simulink model "gm_sampleModel2049_sub"  (R2023a)
settings: Solver=VariableStepAuto  StartTime=0.0  StopTime=10.0  RelTol=1e-3
libraries: simulink x2, hdlsllib x1
settings Model: Creator=user1  LastModifiedBy=user1
settings OptimizationCC: BlockReduction=off  ConditionallyExecuteInputs=off
settings DebuggingCC: InheritedTsInSrcMsg=none

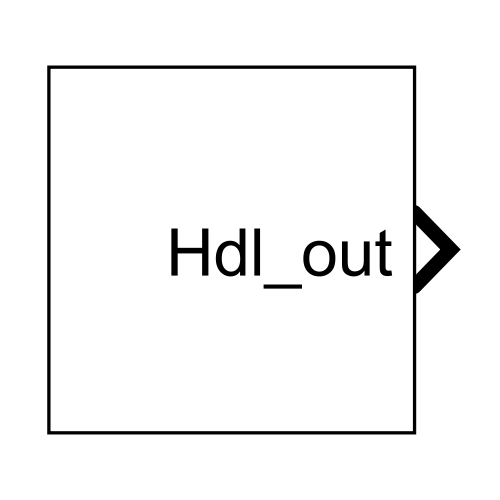
[thumbnail: Simulink's stored preview of the top-level diagram]
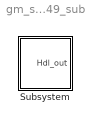
== system gm_sampleModel2049_sub ==
  Subsystem : Subsystem

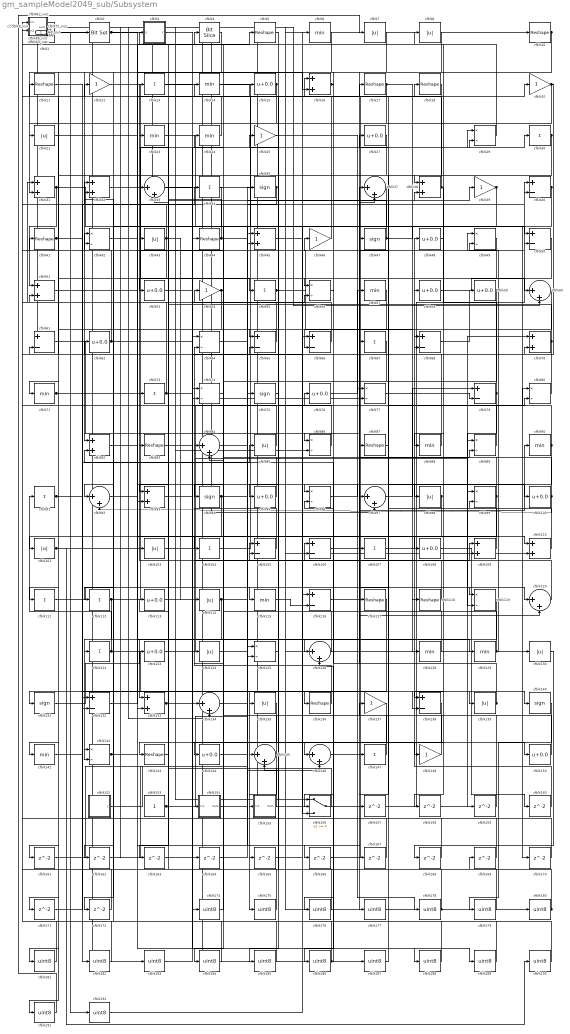
== system gm_sampleModel2049_sub/Subsystem ==
  cfblk1 : simulink/Logic and Bit Operations/Detect Increase  vinit=0.0  OutDataTypeStr=uint8
      settings: LibrarySourceBlock=|
      | hdlsllib/Logic and Bit
      | Operations/Detect
      | Increase
  cfblk{5,10..11,17..18,41,44,83,87,117..118,136,143} (13 alike) : Reshape
  cfblk{15,27,48,53,58..59,62,76,95,100,108,113,123,144,150} (15 alike) : Bias  Bias=0.0  SaturateOnIntegerOverflow=off
  cfblk{7..8,21,43,85,98,101,103,114,124,130,135,139} (13 alike) : Abs  OutDataTypeStr=uint8  SaturateOnIntegerOverflow=off
  cfblk102_inst : Subsystem
  cfblk{13,30,34,55,67,73,91,104,107,111..112,122,147} (13 alike) : Sum  Inputs=+  OutDataTypeStr=uint8
  cfblk{40,50,61,65..66,68,79,105..106,116,132,138} (12 alike) : Sum  Inputs=+-  OutDataTypeStr=uint8
  cfblk{16,31..32,38,45,51,70,82,93,109..110,133} (12 alike) : Sum  OutDataTypeStr=uint8
  cfblk{6,14,23..24,57,71,88,90,115,128..129,141} (12 alike) : MinMax  OutDataTypeStr=uint8
  cfblk{29,42,49,56,64,74,77,80,86,89,96,99,119,125,142} (15 alike) : Product  Inputs=*/  OutDataTypeStr=uint8  RndMeth=Zero  SaturateOnIntegerOverflow=on
  cfblk{12,20,25,39,46,54,137,148} (8 alike) : Gain  OutDataTypeStr=uint8
  cfblk{33,37,60,84,92,97,120,126,134,145..146} (11 alike) : Sum  Inputs=|++  OutDataTypeStr=uint8
  cfblk121_inst : Subsystem
  cfblk127_inst : Subsystem
  cfblk{35,47,75,94,131,140} (6 alike) : Signum
  cfblk152 : Subsystem  mask(Counter Free-Running){NumBits=double(16), tsamp=double(-1)}
      mask prompts: NumBits "Simulink:masks:NumberOfBits_MP"; tsamp "Simulink:masks:SampleTime_MP"
      mask help: Simulink:masks:CounterFreeRunning_MD
  cfblk153 : Constant  OutDataTypeStr=uint8  SampleTime=-1
  cfblk154 : Subsystem
  cfblk155 : Subsystem
  cfblk156 : Switch  OutDataTypeStr=uint8  SaturateOnIntegerOverflow=off  InputSameDT=off
  cfblk{157..172} (16 alike) : Delay  SampleTime=1
  cfblk{174..192} (19 alike) : DataTypeConversion  OutDataTypeStr=uint8  SaturateOnIntegerOverflow=off  RndMeth=Floor
  cfblk19_inst : Subsystem
  cfblk2 : simulink/Logic and Bit Operations/Bit Set  iBit=0
      settings: LibrarySourceBlock=|
      | hdlsllib/Logic and Bit
      | Operations/Bit Set
  cfblk26_inst : Subsystem
  cfblk28_inst : Subsystem
  cfblk3 : Subsystem  mask(Detect Rise Nonnegative){vinit=double(0), InputProcessing=Elements as channels (sample based), OutDataTypeStr=uint8}
      mask prompts: vinit "Simulink:masks:InitialCondition_MP"; InputProcessing "Simulink:masks:InputProcessing_MP"; OutDataTypeStr "Simulink:masks:OutputDataType_MP"
      mask help: Simulink:masks:DetectRiseNonnegative_MD
      mask init:
      | InputProcessing = 'Elements as channels (sample based)';
      | OutDataTypeStr = 'uint8';
      | vinit = double(0);
      mask TypeOptions InputProcessing: Simulink:masks:ColumnsAsChannelsFrameBased | Simulink:masks:ElementsAsChannelsSampleBased
      mask TypeOptions OutDataTypeStr: Simulink:masks:uint8 | Simulink:masks:boolean
      mask Display: fprintf('U >= 0\n&  NOT\nU/z >= 0')
  cfblk36_inst : Subsystem
  cfblk4 : hdlsllib/Logic and Bit Operations/Bit Slice  lidx=7  ridx=0
  cfblk63_inst : Subsystem
  cfblk69_inst : Subsystem
  cfblk72_inst : Subsystem
  cfblk81_inst : Subsystem
  cfblk9_inst : Subsystem
  Hdl_out : Outport  OutDataTypeStr=uint8  SampleTime=1
  wires:
  cfblk1/1 -> cfblk2/1, cfblk192/1
  cfblk10/1 -> cfblk82/1, cfblk177/1
  cfblk100/1 -> cfblk92/2, cfblk14/1
  cfblk101/1 -> cfblk190/1, cfblk46/1
  cfblk102_inst/1(out1) -> cfblk121_inst/1(in1)
  cfblk103/1 -> cfblk76/1
  cfblk104/1 -> cfblk16/1
  cfblk105/1 -> cfblk64/2
  cfblk106/1 -> cfblk20/1
  cfblk107/1 -> cfblk48/1
  cfblk108/1 -> cfblk160/1
  cfblk109/1 -> cfblk27/1
  cfblk11/1 -> cfblk182/1
  cfblk110/1 -> cfblk99/2
  cfblk111/1 -> cfblk119/1
  cfblk112/1 -> cfblk29/2, cfblk142/2, cfblk115/1
  cfblk113/1 -> cfblk109/1
  cfblk114/1 -> cfblk133/1, cfblk39/1
  cfblk115/1 -> cfblk116/2
  cfblk116/1 -> cfblk89/2
  cfblk117/1 -> cfblk131/1
  cfblk118/1 -> cfblk37/1
  cfblk119/1 -> cfblk142/1
  cfblk12/1 -> cfblk55/1
  cfblk120/1 -> cfblk13/1
  cfblk121_inst/1(out1) -> cfblk26_inst/2(in2), cfblk86/2, cfblk159/1
  cfblk122/1 -> cfblk175/1, cfblk91/1
  cfblk123/1 -> cfblk89/1
  cfblk124/1 -> cfblk45/2
  cfblk125/1 -> cfblk105/1
  cfblk126/1 -> cfblk84/2
  cfblk127_inst/1(out1) -> cfblk183/1
  cfblk128/1 -> cfblk45/1
  cfblk129/1 -> cfblk96/2, cfblk49/2
  cfblk13/1 -> cfblk146/1
  cfblk130/1 -> cfblk168/1
  cfblk131/1 -> cfblk123/1
  cfblk132/1 -> cfblk18/1
  cfblk133/1 -> cfblk134/1, cfblk80/2, cfblk30/1
  cfblk134/1 -> cfblk75/1
  cfblk135/1 -> cfblk145/1
  cfblk136/1 -> cfblk84/1
  cfblk137/1 -> cfblk186/1
  cfblk138/1 -> cfblk143/1
  cfblk139/1 -> cfblk97/1, cfblk82/2
  cfblk14/1 -> cfblk170/1
  cfblk140/1 -> cfblk179/1
  cfblk141/1 -> cfblk85/1
  cfblk142/1 -> cfblk166/1, cfblk165/1
  cfblk143/1 -> cfblk113/1
  cfblk144/1 -> cfblk106/1
  cfblk145/1 -> cfblk61/2, cfblk155/1(In1)
  cfblk146/1 -> cfblk90/1
  cfblk147/1 -> cfblk81_inst/2(in2)
  cfblk148/1 -> cfblk58/1
  cfblk15/1 -> cfblk31/2, cfblk181/1, Hdl_out/1
  cfblk150/1 -> cfblk83/1
  cfblk152/1(y) -> cfblk49/1
  cfblk153/1 -> cfblk35/1, cfblk154/1(In1)
  cfblk154/1(Out1) -> cfblk80/1
  cfblk155/1(Out1) -> cfblk103/1
  cfblk156/1 -> cfblk23/1
  cfblk157/1 -> cfblk40/1
  cfblk158/1 -> cfblk70/1
  cfblk159/1 -> cfblk99/1
  cfblk16/1 -> cfblk66/2, cfblk156/2
  cfblk160/1 -> cfblk68/1
  cfblk161/1 -> cfblk74/1
  cfblk162/1 -> cfblk38/2
  cfblk163/1 -> cfblk64/1
  cfblk164/1 -> cfblk146/2
  cfblk165/1 -> cfblk106/2
  cfblk166/1 -> cfblk120/2
  cfblk167/1 -> cfblk105/2
  cfblk168/1 -> cfblk102_inst/1(in1)
  cfblk169/1 -> cfblk63_inst/2(in2)
  cfblk17/1 -> cfblk53/1, cfblk120/1
  cfblk170/1 -> cfblk33/2
  cfblk171/1 -> cfblk132/1
  cfblk172/1 -> cfblk121_inst/2(in2)
  cfblk174/1 -> cfblk124/1
  cfblk175/1 -> cfblk3/1(U)
  cfblk176/1 -> cfblk72_inst/1(in1)
  cfblk177/1 -> cfblk67/1
  cfblk178/1 -> cfblk43/1, cfblk54/1
  cfblk179/1 -> cfblk25/1
  cfblk18/1 -> cfblk38/1
  cfblk180/1 -> cfblk17/1, cfblk145/2, cfblk169/1
  cfblk181/1 -> cfblk19_inst/1(in1)
  cfblk182/1 -> cfblk19_inst/2(in2)
  cfblk183/1 -> cfblk44/1
  cfblk184/1 -> cfblk127_inst/1(in1)
  cfblk185/1 -> cfblk127_inst/2(in2)
  cfblk186/1 -> cfblk36_inst/2(in2), cfblk32/1, cfblk126/2
  cfblk187/1 -> cfblk137/1
  cfblk188/1 -> cfblk81_inst/1(in1)
  cfblk189/1 -> cfblk42/1
  cfblk19_inst/1(out1) -> cfblk180/1
  cfblk190/1 -> cfblk42/2
  cfblk191/1 -> cfblk7/1
  cfblk192/1 -> cfblk6/1
  cfblk2/1 -> cfblk16/2, cfblk140/1
  cfblk20/1 -> cfblk70/2, cfblk65/1
  cfblk21/1 -> cfblk110/1
  cfblk23/1 -> cfblk128/1
  cfblk24/1 -> cfblk63_inst/1(in1)
  cfblk25/1 -> cfblk178/1
  cfblk26_inst/1(out1) -> cfblk61/1
  cfblk27/1 -> cfblk71/1
  cfblk28_inst/1(out1) -> cfblk77/2, cfblk164/1
  cfblk29/1 -> cfblk28_inst/1(in1)
  cfblk3/1(Y) -> cfblk174/1
  cfblk30/1 -> cfblk92/1, cfblk147/1
  cfblk31/1 -> cfblk51/1, cfblk77/1
  cfblk32/1 -> cfblk125/1
  cfblk33/1 -> cfblk74/2
  cfblk34/1 -> cfblk172/1
  cfblk35/1 -> cfblk32/2, cfblk1/1
  cfblk36_inst/1(out1) -> cfblk97/2
  cfblk37/1 -> cfblk162/1
  cfblk38/1 -> cfblk102_inst/2(in2), cfblk158/1
  cfblk39/1 -> cfblk117/1, cfblk104/1
  cfblk4/1 -> cfblk21/1
  cfblk40/1 -> cfblk156/3, cfblk144/1, cfblk148/1, cfblk88/1
  cfblk41/1 -> cfblk139/1, cfblk73/1
  cfblk42/1 -> cfblk188/1
  cfblk43/1 -> cfblk93/1, cfblk72_inst/2(in2), cfblk133/2, cfblk114/1
  cfblk44/1 -> cfblk36_inst/1(in1), cfblk167/1
  cfblk45/1 -> cfblk29/1
  cfblk46/1 -> cfblk12/1
  cfblk47/1 -> cfblk9_inst/2(in2), cfblk50/1
  cfblk48/1 -> cfblk138/1
  cfblk49/1 -> cfblk184/1
  cfblk5/1 -> cfblk185/1
  cfblk50/1 -> cfblk101/1
  cfblk51/1 -> cfblk100/1
  cfblk53/1 -> cfblk150/1
  cfblk54/1 -> cfblk93/2, cfblk24/1
  cfblk55/1 -> cfblk37/2, cfblk118/1
  cfblk56/1 -> cfblk126/1
  cfblk57/1 -> cfblk161/1
  cfblk58/1 -> cfblk60/1
  cfblk59/1 -> cfblk94/1, cfblk135/1, cfblk108/1
  cfblk6/1 -> cfblk191/1
  cfblk60/1 -> cfblk163/1
  cfblk61/1 -> cfblk116/1
  cfblk62/1 -> cfblk69_inst/2(in2), cfblk26_inst/1(in1), cfblk56/2
  cfblk63_inst/1(out1) -> cfblk110/2, cfblk10/1
  cfblk64/1 -> cfblk40/2
  cfblk65/1 -> cfblk9_inst/1(in1)
  cfblk66/1 -> cfblk11/1
  cfblk67/1 -> cfblk176/1
  cfblk68/1 -> cfblk59/1
  cfblk69_inst/1(out1) -> cfblk130/1
  cfblk7/1 -> cfblk112/1
  cfblk70/1 -> cfblk65/2, cfblk33/1
  cfblk71/1 -> cfblk5/1, cfblk141/1
  cfblk72_inst/1(out1) -> cfblk187/1, cfblk134/2
  cfblk73/1 -> cfblk31/1, cfblk86/1, cfblk125/2
  cfblk74/1 -> cfblk4/1
  cfblk75/1 -> cfblk95/1
  cfblk76/1 -> cfblk57/1
  cfblk77/1 -> cfblk79/2
  cfblk79/1 -> cfblk8/1, cfblk119/2
  cfblk8/1 -> cfblk56/1
  cfblk80/1 -> cfblk28_inst/2(in2)
  cfblk81_inst/1(out1) -> cfblk60/2
  cfblk82/1 -> cfblk96/1
  cfblk83/1 -> cfblk189/1
  cfblk84/1 -> cfblk87/1
  cfblk85/1 -> cfblk69_inst/1(in1)
  cfblk86/1 -> cfblk15/1
  cfblk87/1 -> cfblk157/1
  cfblk88/1 -> cfblk51/2
  cfblk89/1 -> cfblk47/1
  cfblk9_inst/1(out1) -> cfblk156/1
  cfblk90/1 -> cfblk68/2, cfblk109/2, cfblk107/1
  cfblk91/1 -> cfblk138/2, cfblk34/1
  cfblk92/1 -> cfblk129/1
  cfblk93/1 -> cfblk66/1
  cfblk94/1 -> cfblk50/2, cfblk111/1
  cfblk95/1 -> cfblk41/1
  cfblk96/1 -> cfblk98/1
  cfblk97/1 -> cfblk79/1
  cfblk98/1 -> cfblk171/1, cfblk122/1
  cfblk99/1 -> cfblk62/1, cfblk136/1, cfblk132/2

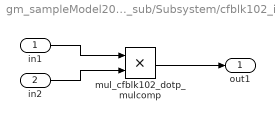
== system gm_sampleModel2049_sub/Subsystem/cfblk102_inst ==
  in1 : Inport  OutDataTypeStr=uint8  SampleTime=1
  in2 : Inport  Port=2  OutDataTypeStr=uint8  SampleTime=1
  mul_cfblk102_dotp_mulcomp : Product  Inputs=**  OutDataTypeStr=uint8  SampleTime=1
  out1 : Outport  OutDataTypeStr=uint8  SampleTime=1
  wires:
  in1/1 -> mul_cfblk102_dotp_mulcomp/1
  in2/1 -> mul_cfblk102_dotp_mulcomp/2
  mul_cfblk102_dotp_mulcomp/1 -> out1/1

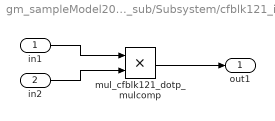
== system gm_sampleModel2049_sub/Subsystem/cfblk121_inst ==
  in1 : Inport  OutDataTypeStr=uint8  SampleTime=1
  in2 : Inport  Port=2  OutDataTypeStr=uint8  SampleTime=1
  mul_cfblk121_dotp_mulcomp : Product  Inputs=**  OutDataTypeStr=uint8  SampleTime=1
  out1 : Outport  OutDataTypeStr=uint8  SampleTime=1
  wires:
  in1/1 -> mul_cfblk121_dotp_mulcomp/1
  in2/1 -> mul_cfblk121_dotp_mulcomp/2
  mul_cfblk121_dotp_mulcomp/1 -> out1/1

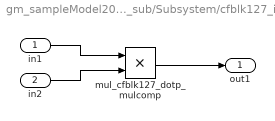
== system gm_sampleModel2049_sub/Subsystem/cfblk127_inst ==
  in1 : Inport  OutDataTypeStr=uint8  SampleTime=1
  in2 : Inport  Port=2  OutDataTypeStr=uint8  SampleTime=1
  mul_cfblk127_dotp_mulcomp : Product  Inputs=**  OutDataTypeStr=uint8  SampleTime=1
  out1 : Outport  OutDataTypeStr=uint8  SampleTime=1
  wires:
  in1/1 -> mul_cfblk127_dotp_mulcomp/1
  in2/1 -> mul_cfblk127_dotp_mulcomp/2
  mul_cfblk127_dotp_mulcomp/1 -> out1/1

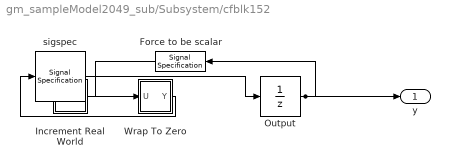
== system gm_sampleModel2049_sub/Subsystem/cfblk152 ==
  Force to be scalar : SignalSpecification  DisableCoverage=on  Dimensions=1
  Increment Real World : Subsystem  mask(Real World Value Increment){}
      mask help: Simulink:masks:RealWorldValueIncrement_MD
      mask Display: disp('V++')
  Output : UnitDelay  InitialCondition=0.0  SampleTime=tsamp  HasFrameUpgradeWarning=on
  Wrap To Zero : Subsystem  mask(Wrap To Zero){Threshold=double(65535)}
      mask prompts: Threshold "Simulink:masks:Threshold_MP"
      mask help: Simulink:masks:WrapToZero_MD
  sigspec : SignalSpecification  OutDataTypeStr=uint16  Dimensions=1
  y : Outport  SampleTime=1
  wires:
  Force to be scalar/1 -> Increment Real World/1(u)
  Increment Real World/1(y) -> Wrap To Zero/1(U)
  Output/1 -> Force to be scalar/1, y/1
  Wrap To Zero/1(Y) -> sigspec/1
  sigspec/1 -> Output/1

== system gm_sampleModel2049_sub/Subsystem/cfblk154 ==
  In1 : Inport  OutDataTypeStr=uint8  PortDimensions=1  SampleTime=1
  Out1 : Outport  SampleTime=1
  wires:
  In1/1 -> Out1/1

== system gm_sampleModel2049_sub/Subsystem/cfblk155 ==
  In1 : Inport  OutDataTypeStr=uint8  PortDimensions=1  SampleTime=1
  Out1 : Outport  SampleTime=1
  wires:
  In1/1 -> Out1/1

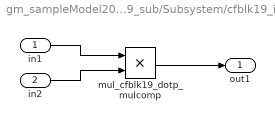
== system gm_sampleModel2049_sub/Subsystem/cfblk19_inst ==
  in1 : Inport  OutDataTypeStr=uint8  SampleTime=1
  in2 : Inport  Port=2  OutDataTypeStr=uint8  SampleTime=1
  mul_cfblk19_dotp_mulcomp : Product  Inputs=**  OutDataTypeStr=uint8  SampleTime=1
  out1 : Outport  OutDataTypeStr=uint8  SampleTime=1
  wires:
  in1/1 -> mul_cfblk19_dotp_mulcomp/1
  in2/1 -> mul_cfblk19_dotp_mulcomp/2
  mul_cfblk19_dotp_mulcomp/1 -> out1/1

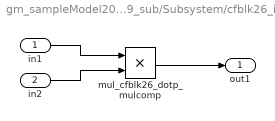
== system gm_sampleModel2049_sub/Subsystem/cfblk26_inst ==
  in1 : Inport  OutDataTypeStr=uint8  SampleTime=1
  in2 : Inport  Port=2  OutDataTypeStr=uint8  SampleTime=1
  mul_cfblk26_dotp_mulcomp : Product  Inputs=**  OutDataTypeStr=uint8  SampleTime=1
  out1 : Outport  OutDataTypeStr=uint8  SampleTime=1
  wires:
  in1/1 -> mul_cfblk26_dotp_mulcomp/1
  in2/1 -> mul_cfblk26_dotp_mulcomp/2
  mul_cfblk26_dotp_mulcomp/1 -> out1/1

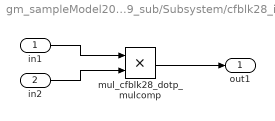
== system gm_sampleModel2049_sub/Subsystem/cfblk28_inst ==
  in1 : Inport  OutDataTypeStr=uint8  SampleTime=1
  in2 : Inport  Port=2  OutDataTypeStr=uint8  SampleTime=1
  mul_cfblk28_dotp_mulcomp : Product  Inputs=**  OutDataTypeStr=uint8  SampleTime=1
  out1 : Outport  OutDataTypeStr=uint8  SampleTime=1
  wires:
  in1/1 -> mul_cfblk28_dotp_mulcomp/1
  in2/1 -> mul_cfblk28_dotp_mulcomp/2
  mul_cfblk28_dotp_mulcomp/1 -> out1/1

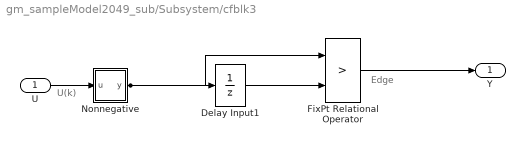
== system gm_sampleModel2049_sub/Subsystem/cfblk3 ==
  note: U(k)
  note: Edge
  U : Inport  OutDataTypeStr=uint8  SampleTime=1
  Delay Input1 : UnitDelay  Description=Store in Global RAM  DisableCoverage=on  InitialCondition=vinit  SampleTime=-1  HasFrameUpgradeWarning=on
  FixPt Relational Operator : RelationalOperator  Operator=>  OutDataTypeStr=fixdt(0, 8)  ZeroCross=off  InputSameDT=off
  Nonnegative : Subsystem  mask(Compare To Zero){relop=>=, OutDataTypeStr=boolean, ZeroCross=off}
      mask prompts: relop "Simulink:masks:Operator_MP"; OutDataTypeStr "Simulink:masks:OutputDataType_MP"; ZeroCross "Simulink:masks:EnableZerocrossingDetection_MP"
      mask help: Simulink:masks:CompareToZero_MD
      mask init:
      | OutDataTypeStr = 'boolean';
      | ZeroCross = 'off';
      | blkName = 'sampleModel2049_sub/Subsystem/cfblk3/Nonnegative';
      | relop = '>=';
      | setValue = 'boolean';
      mask TypeOptions relop: == | ~= | < | <= | >= | >
      mask TypeOptions OutDataTypeStr: Simulink:masks:uint8 | Simulink:masks:boolean
      mask Callback ZeroCross: sl('zeroCrossEnable', gcbh);
      mask Display: disp([relop,' 0'])
  Y : Outport  SampleTime=1
  wires:
  U/1 -> Nonnegative/1(u)
  Delay Input1/1 -> FixPt Relational Operator/2
  FixPt Relational Operator/1 -> Y/1
  Nonnegative/1(y) -> FixPt Relational Operator/1, Delay Input1/1

== system gm_sampleModel2049_sub/Subsystem/cfblk36_inst ==
  in1 : Inport  OutDataTypeStr=uint8  SampleTime=1
  in2 : Inport  Port=2  OutDataTypeStr=uint8  SampleTime=1
  mul_cfblk36_dotp_mulcomp : Product  Inputs=**  OutDataTypeStr=uint8  SampleTime=1
  out1 : Outport  OutDataTypeStr=uint8  SampleTime=1
  wires:
  in1/1 -> mul_cfblk36_dotp_mulcomp/1
  in2/1 -> mul_cfblk36_dotp_mulcomp/2
  mul_cfblk36_dotp_mulcomp/1 -> out1/1

== system gm_sampleModel2049_sub/Subsystem/cfblk63_inst ==
  in1 : Inport  OutDataTypeStr=uint8  SampleTime=1
  in2 : Inport  Port=2  OutDataTypeStr=uint8  SampleTime=1
  mul_cfblk63_dotp_mulcomp : Product  Inputs=**  OutDataTypeStr=uint8  SampleTime=1
  out1 : Outport  OutDataTypeStr=uint8  SampleTime=1
  wires:
  in1/1 -> mul_cfblk63_dotp_mulcomp/1
  in2/1 -> mul_cfblk63_dotp_mulcomp/2
  mul_cfblk63_dotp_mulcomp/1 -> out1/1

== system gm_sampleModel2049_sub/Subsystem/cfblk69_inst ==
  in1 : Inport  OutDataTypeStr=uint8  SampleTime=1
  in2 : Inport  Port=2  OutDataTypeStr=uint8  SampleTime=1
  mul_cfblk69_dotp_mulcomp : Product  Inputs=**  OutDataTypeStr=uint8  SampleTime=1
  out1 : Outport  OutDataTypeStr=uint8  SampleTime=1
  wires:
  in1/1 -> mul_cfblk69_dotp_mulcomp/1
  in2/1 -> mul_cfblk69_dotp_mulcomp/2
  mul_cfblk69_dotp_mulcomp/1 -> out1/1

== system gm_sampleModel2049_sub/Subsystem/cfblk72_inst ==
  in1 : Inport  OutDataTypeStr=uint8  SampleTime=1
  in2 : Inport  Port=2  OutDataTypeStr=uint8  SampleTime=1
  mul_cfblk72_dotp_mulcomp : Product  Inputs=**  OutDataTypeStr=uint8  SampleTime=1
  out1 : Outport  OutDataTypeStr=uint8  SampleTime=1
  wires:
  in1/1 -> mul_cfblk72_dotp_mulcomp/1
  in2/1 -> mul_cfblk72_dotp_mulcomp/2
  mul_cfblk72_dotp_mulcomp/1 -> out1/1

== system gm_sampleModel2049_sub/Subsystem/cfblk81_inst ==
  in1 : Inport  OutDataTypeStr=uint8  SampleTime=1
  in2 : Inport  Port=2  OutDataTypeStr=uint8  SampleTime=1
  mul_cfblk81_dotp_mulcomp : Product  Inputs=**  OutDataTypeStr=uint8  SampleTime=1
  out1 : Outport  OutDataTypeStr=uint8  SampleTime=1
  wires:
  in1/1 -> mul_cfblk81_dotp_mulcomp/1
  in2/1 -> mul_cfblk81_dotp_mulcomp/2
  mul_cfblk81_dotp_mulcomp/1 -> out1/1

== system gm_sampleModel2049_sub/Subsystem/cfblk9_inst ==
  in1 : Inport  OutDataTypeStr=uint8  SampleTime=1
  in2 : Inport  Port=2  OutDataTypeStr=uint8  SampleTime=1
  mul_cfblk9_dotp_mulcomp : Product  Inputs=**  OutDataTypeStr=uint8  SampleTime=1
  out1 : Outport  OutDataTypeStr=uint8  SampleTime=1
  wires:
  in1/1 -> mul_cfblk9_dotp_mulcomp/1
  in2/1 -> mul_cfblk9_dotp_mulcomp/2
  mul_cfblk9_dotp_mulcomp/1 -> out1/1

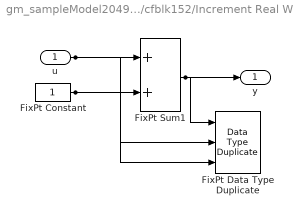
== system gm_sampleModel2049_sub/Subsystem/cfblk152/Increment Real World ==
  u : Inport  OutDataTypeStr=uint16  SampleTime=1
  FixPt Constant : Constant  DisableCoverage=on  OutDataTypeStr=Inherit: Inherit via back propagation  SampleTime=-1
  FixPt Data Type Duplicate : DataTypeDuplicate  DisableCoverage=on  NumInputPorts=3
  FixPt Sum1 : Sum  InputSameDT=on  OutDataTypeStr=Inherit: Inherit via back propagation  LockScale=on
  y : Outport  SampleTime=1
  wires:
  u/1 -> FixPt Sum1/1, FixPt Data Type Duplicate/2
  FixPt Constant/1 -> FixPt Sum1/2, FixPt Data Type Duplicate/3
  FixPt Sum1/1 -> FixPt Data Type Duplicate/1, y/1

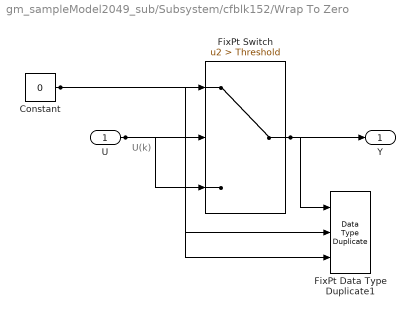
== system gm_sampleModel2049_sub/Subsystem/cfblk152/Wrap To Zero ==
  note: U(k)
  U : Inport  OutDataTypeStr=uint16  SampleTime=1
  Constant : Constant  DisableCoverage=on  Value=0  OutDataTypeStr=Inherit: Inherit via back propagation  SampleTime=-1
  FixPt Data Type Duplicate1 : DataTypeDuplicate  DisableCoverage=on  NumInputPorts=3
  FixPt Switch : Switch  Criteria=u2 > Threshold  Threshold=Threshold  OutDataTypeStr=Inherit: Inherit via back propagation  ZeroCross=off  SaturateOnIntegerOverflow=off  InputSameDT=off
  Y : Outport  SampleTime=1
  wires:
  U/1 -> FixPt Switch/3, FixPt Switch/2, FixPt Data Type Duplicate1/2
  Constant/1 -> FixPt Switch/1, FixPt Data Type Duplicate1/3
  FixPt Switch/1 -> FixPt Data Type Duplicate1/1, Y/1

== system gm_sampleModel2049_sub/Subsystem/cfblk3/Nonnegative ==
  u : Inport  OutDataTypeStr=uint8  SampleTime=1
  Compare : RelationalOperator  OutDataTypeStr=boolean  ZeroCross=off
  Constant : Constant  DisableCoverage=on  Value=0  OutDataTypeStr=Inherit: Inherit via back propagation  SampleTime=-1  PreserveConstantTs=on
  y : Outport  SampleTime=1
  wires:
  u/1 -> Compare/1
  Compare/1 -> y/1
  Constant/1 -> Compare/2
